simulink model "FOC_ControlState_ref"  (R2022b)
settings: Solver=FixedStepDiscrete  StartTime=0.0  StopTime=160  FixedStep=0.000005  RelTol=1e-3  EnableMultiTasking=on
settings Model: RequirementInfo={} %GIDa_fe9045fd_0412_4b6e_8206_617cc20e6fde  FPTRunName=Active  Creator=ts  LastModifiedBy=hufnagelde
settings SolverCC: AlgebraicLoopSolver=TrustRegion  PositivePriorityOrder=on  AutoInsertRateTranBlk=on
settings DataIOCC: SaveOutput=off  SignalLogging=off  DSMLogging=off  SaveTime=off
settings OptimizationCC: DefaultParameterBehavior=Inlined  UseDivisionForNetSlopeComputation=on  GainParamInheritBuiltInType=on  UseFloatMulNetSlope=on  DefaultUnderspecifiedDataType=single  UseSpecifiedMinMax=on  InlineInvariantSignals=on  PassReuseOutputArgsAs=Individual arguments  ZeroExternalMemoryAtStartup=off  ZeroInternalMemoryAtStartup=off  NoFixptDivByZeroProtection=on  EfficientFloat2IntCast=on  LifeSpan=1  MaxStackSize=64  OptimizeBlockOrder=speed  DifferentSizesBufferReuse=on  EfficientTunableParamExpr=on
settings DebuggingCC: UnconnectedInputMsg=warning  UnconnectedOutputMsg=warning  UnconnectedLineMsg=warning  BusObjectLabelMismatch=error  AllowSymbolicDim=off  SFUnexpectedBacktrackingDiag=warning  SFNoUnconditionalDefaultTransitionDiag=warning  SFExecutionAtInitializationDiag=none  SFMachineParentedDataDiag=warning  ArithmeticOperatorsInVariantConditions=warning
settings HardwareCC: ProdBitPerPointer=32  ProdBitPerSizeT=32  ProdBitPerPtrDiffT=32  ProdLargestAtomicInteger=Long  ProdLargestAtomicFloat=Double  ProdWordSize=32  ProdLongLongMode=on  ProdHWDeviceType=ARM Compatible->ARM Cortex-R  HardwareBoardFeatureSet=SoCBlockset
settings ModelReferenceCC: EnableRefExpFcnMdlSchedulingChecks=on
settings SFSimCC: SimGenImportedTypeDefs=on  MATLABDynamicMemAlloc=off
settings RTWCC: Description=Embedded Coder  SystemTargetFile=ert.tlc  GenCodeOnly=on  TemplateMakefile=ert_default_tmf  GenerateReport=on  BuildConfiguration=Faster Runs  IncludeHyperlinkInReport=on  LaunchReport=on  GenerateTraceInfo=on  GenerateTraceReport=on  GenerateTraceReportSl=on  GenerateTraceReportSf=on  GenerateTraceReportEml=on  GenerateCodeMetricsReport=on  CheckMdlBeforeBuild=Warning  DLArmComputeVersion=19.05
settings CodeAppCC: ForceParamTrailComments=on  IgnoreCustomStorageClasses=off  OperatorAnnotations=on  SimulinkDataObjDesc=on  SFDataObjDesc=on  MATLABFcnDesc=on  CustomSymbolStrGlobalVar=rt$M$R$N  CustomSymbolStrType=$N$M$R_t  CustomSymbolStrFcn=$N$M$F  CustomSymbolStrMacro=$N$M  InsertBlockDesc=on  StateflowObjectComments=on  MATLABSourceComments=on  EnableCustomComments=on  ReqsInCode=on
settings ERTTargetCC: TargetLangStandard=C99 (ISO)  CodeReplacementLibrary=GNU C99 extensions  MultiwordLength=2048  IncludeMdlTerminateFcn=off  CombineSignalStateStructs=on  SuppressErrorStatus=on  IncludeFileDelimiter=UseQuote  SupportAbsoluteTime=off  CodeInterfacePackaging=Reusable function  SupportNonFinite=off  RemoveResetFunc=off  InlinedParameterPlacement=NonHierarchical  MultiInstanceErrorCode=Warning  RootIOFormat=Part of model data structure  ERTCustomFileTemplate=example_file_process.tlc  GlobalDataDefinition=InSourceFile  GlobalDataReference=InSourceFile  ERTFilePackagingFormat=CompactWithDataFile  SuppressUnreachableDefaultCases=off
settings ConfigComp: CovScope=ReferencedModels  CovSaveName=covdata_rollAP  CovMetricSettings=dcmtrwe  CovHTMLOptions=-sRT=1 -aTS=1 -bRG=1 -bTC=1 -hTR=1 -nFC=0 -scm=1 -bcm=1 -xEv=0  CovSaveCumulativeToWorkspaceVar=on  CovSaveSingleToWorkspaceVar=on  CovCumulativeVarName=covCumulativeData_rollAP  CovReportOnPause=off  CovExternalEMLEnable=off  CovSFcnEnable=off

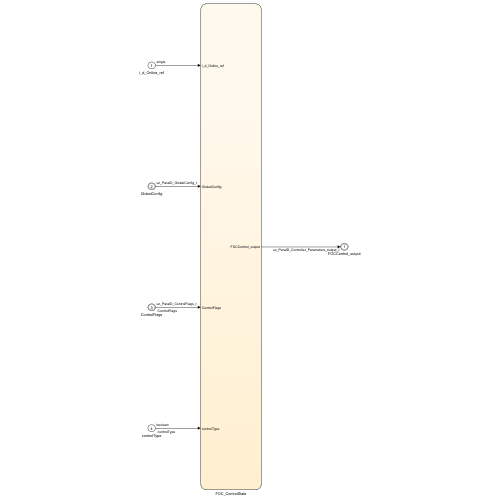
[thumbnail: Simulink's stored preview of the top-level diagram]
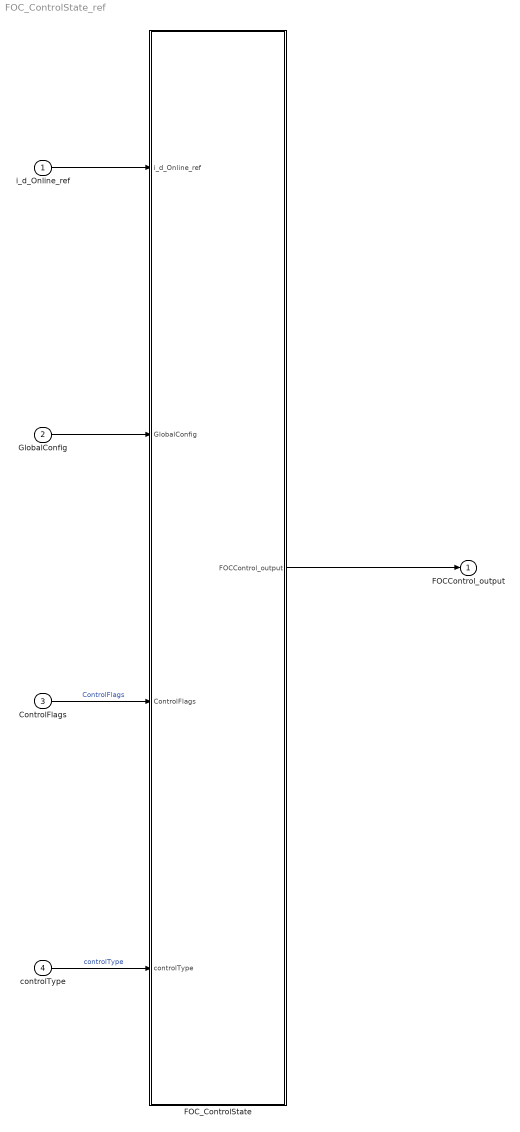
== system FOC_ControlState_ref ==
  i_d_Online_ref : Inport  OutDataTypeStr=single  PortDimensions=1  SampleTime=[5.0000000000000002e-05,0]
  GlobalConfig : Inport  Port=2  OutDataTypeStr=Bus: uz_ParaID_GlobalConfig_t  PortDimensions=1  SampleTime=[5.0000000000000002e-05,0]  BusOutputAsStruct=on
  ControlFlags : Inport  Port=3  OutDataTypeStr=Bus: uz_ParaID_ControlFlags_t  PortDimensions=1  SampleTime=[5.0000000000000002e-05,0]  BusOutputAsStruct=on
  controlType : Inport  Port=4  OutDataTypeStr=boolean  PortDimensions=1  SampleTime=[5.0000000000000002e-05,0]
  FOC_ControlState : Stateflow chart  TreatAsAtomicUnit=on
  FOCControl_output : Outport  OutDataTypeStr=Bus: uz_ParaID_Controller_Parameters_output_t  PortDimensions=1  SampleTime=[5.0000000000000002e-05,0]  BusOutputAsStruct=on
  wires:
  i_d_Online_ref/1 -> FOC_ControlState/1(i_d_Online_ref)
  GlobalConfig/1 -> FOC_ControlState/2(GlobalConfig)
  ControlFlags/1 -> FOC_ControlState/3(ControlFlags)  "ControlFlags"
  controlType/1 -> FOC_ControlState/4(controlType)  "controlType"
  FOC_ControlState/1(FOCControl_output) -> FOCControl_output/1

== stateflow chart FOC_ControlState_ref/FOC_ControlState ==
  settings: updateMethod=DISCRETE  sampleTime=1/d_f_states
  note: Control-States
  state FOC_ControlState
    entry:
    FOCControl_output.activeState = uint16(600);
    initParams;
    during:
    note: FOC current control
    state FOCcurrentControl 	%state 140
      entry:
      FOCControl_output.activeState = uint16(610);
      FOCControl_output.enableFOC_current=boolean(1);
      counter = uint32(1);
      during:
      FOCControl_output.i_dq_ref.q=GlobalConfig.i_dq_ref.q;
      FOCControl_output.i_dq_ref.d=GlobalConfig.i_dq_ref.d+i_d_Online_ref;
      exit:
      counter = uint32(1);
      FOCControl_output.enableFOC_current=boolean(0);
    state FOCdecider
      entry:
    note: FOC speed control
    note: change speed with sinusoidal trajectory in 0.2 sec
    state FOCspeed_speedChange 	%state 13.0
      entry:
      FOCControl_output.activeState = uint16(620);
      FOCControl_output.enableFOC_speed=boolean(1);
      counter = uint32(1);
      during:
      FOCControl_output.i_dq_ref.d = i_d_Online_ref+GlobalConfig.i_dq_ref.d;
      n_filt = single((single(counter)*GlobalConfig.sampleTimeISR*5)-....
      1/(2*pi)*sin(2*pi*single(counter)*GlobalConfig.sampleTimeISR*5));
      FOCControl_output.n_ref_FOC=((GlobalConfig.n_ref-n_ref_old)*n_filt)+n_ref_old;
      counter = counter + 1;
      exit:
      counter = uint32(1);
    state FOCspeed_constantSpeed 		%state 13.1
      entry:
      FOCControl_output.activeState = uint16(621);
      n_ref_old = GlobalConfig.n_ref;
      during:
      FOCControl_output.n_ref_FOC=GlobalConfig.n_ref;
      FOCControl_output.i_dq_ref.d=GlobalConfig.i_dq_ref.d +i_d_Online_ref;
      exit:
      counter = uint32(1);
      FOCControl_output.enableFOC_speed=boolean(0);
      note: constant speed
    (default) -> FOCdecider
    FOCdecider -> FOCcurrentControl 	%state 140 [order 1] : [controlType==0]
    FOCdecider -> FOCspeed_speedChange 	%state 13.0 [order 2] : [controlType==1]
    FOCspeed_constantSpeed 		%state 13.1 -> FOCspeed_speedChange 	%state 13.0 : [GlobalConfig.n_ref~=n_ref_old]
    FOCspeed_speedChange 	%state 13.0 -> FOCspeed_constantSpeed 		%state 13.1 : after(0.2,sec)
  state Waiting
    entry:
    %wait for activation of
    %FOCcontrol
    %donothing
  note: ---
  Waiting -> FOC_ControlState : [GlobalConfig.Reset==0 && ControlFlags.finished_all_Offline_states==1]
  (default) -> Waiting
  FOC_ControlState -> Waiting : [GlobalConfig.Reset==1]
  data: n_ref_old local; n_filt local; i_d_R_online local; counter local; FOCControl_output output Bus: uz_ParaID_Controller_Parameters_output_t; J local; measArray1 local; d local; i_d_Online_ref input; GlobalConfig input Bus: uz_ParaID_GlobalConfig_t; ControlFlags input Bus: uz_ParaID_ControlFlags_t; controlType input
  function initParams:
    | function initParams
    | 
    | % initialize variables
    | n_filt              = single(0.0);
    | n_ref_old           = single(0.0);
    | counter 			= uint32(1);
    | measArray1			= single(zeros(1024,1));
    | i_d_R_online        = single(0.0);
    | d        			= single(zeros(2048,1));
    | J 					= single(zeros(2048,2));
    | 
    | %Outputs
    | FOCControl_output.Ki_n_out          = single(GlobalConfig.Ki_n);
    | FOCControl_output.Ki_iq_out         = single(GlobalConfig.Ki_iq);
    | FOCControl_output.Ki_id_out         = single(GlobalConfig.Ki_id);
    | FOCControl_output.Kp_n_out          = single(GlobalConfig.Kp_n);
    | FOCControl_output.Kp_iq_out         = single(GlobalConfig.Kp_iq);
    | FOCControl_output.Kp_id_out         = single(GlobalConfig.Kp_id);
    | FOCControl_output.n_ref_FOC         = single(0.0);
    | FOCControl_output.M_ref_FOC      	= single(0.0);
    | FOCControl_output.i_dq_ref.d        = single(0.0);
    | FOCControl_output.i_dq_ref.q        = single(0.0);
    | FOCControl_output.i_dq_ref.zero      = single(0.0);
    | FOCControl_output.enableFOC_speed   = boolean(0);
    | FOCControl_output.enableFOC_current	= boolean(0);
    | FOCControl_output.resetIntegrator   = boolean(0);
    | FOCControl_output.activeState       = uint16(0);
    | 
    | end
